simulink model "train"  (Simulink 7.9)
settings: Solver=ode45  SolverMode=SingleTasking  StartTime=0.0  StopTime=1000  RelTol=1e-3  AbsTol=1e-6
undefined symbols (not defined in the file): g, k, M1, M2, mu
settings Model: Creator=Rick  LastModifiedBy=Rick
settings DataIOCC: LimitDataPoints=off
settings OptimizationCC: BlockReduction=off  BooleanDataType=off
settings DebuggingCC: SaveWithParameterizedLinksMsg=none  SignalResolutionControl=TryResolveAllWithWarning  SolverPrmCheckMsg=none  MultiTaskDSMMsg=warning  MultiTaskCondExecSysMsg=none  StrictBusMsg=None
settings HardwareCC: TargetUnknown=on
settings RTWCC: IncludeERTFirstTime=on

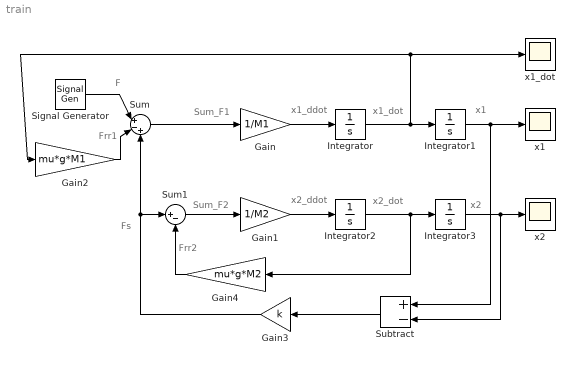
== system train ==
  note: Sum_F1
  note: Sum_F2
  note: x1_ddot
  note: x1_dot
  note: x1
  note: x2_ddot
  note: x2_dot
  note: x2
  note: F
  note: Frr1
  note: Fs
  note: Frr2
  Gain : Gain  Gain=1/M1
  Gain1 : Gain  Gain=1/M2
  Gain2 : Gain  Gain=mu*g*M1
  Gain3 : Gain  Gain=k
  Gain4 : Gain  Gain=mu*g*M2
  Integrator{,1..3} (4 alike) : Integrator
  Signal Generator : SignalGenerator  WaveForm=square  Amplitude=-1  Frequency=0.001
  Subtract : Sum  Inputs=+-
  Sum : Sum  Inputs=|+-+
  Sum1 : Sum  Inputs=|+-
  x1 : Scope
  x1_dot : Scope
      settings: SaveName=ScopeData2
  x2 : Scope
  wires:
  Sum/1 -> Gain/1
  Sum1/1 -> Gain1/1
  Gain/1 -> Integrator/1
  Integrator/1 -> Integrator1/1, Gain2/1, x1_dot/1
  Integrator1/1 -> x1/1, Subtract/1
  Integrator2/1 -> Integrator3/1, Gain4/1
  Integrator3/1 -> x2/1, Subtract/2
  Gain1/1 -> Integrator2/1
  Signal Generator/1 -> Sum/1
  Gain2/1 -> Sum/2
  Subtract/1 -> Gain3/1
  Gain3/1 -> Sum/3, Sum1/1
  Gain4/1 -> Sum1/2
